simulink model "bh_4bar_model_matrix_VEL_ANALYSIS"  (R2020b)
settings: Solver=ode45  StartTime=0.0  StopTime=2.0944  MaxStep=0.1  RelTol=1e-5  EnableMultiTasking=on
values from neighbouring files (symbols this model uses):
  N = length(THE_DEG_ANG_VEC)    [bh_4bar_kin_z_analysis_CLS.m]
  X = my_stuff_T.theta_deg_vec    [bh_4bar_kin_z_analysis_CLS.m]
undefined symbols (not defined in the file or in its folder): H, my_L1, my_L2, my_L3, theta_0_rad, theta_dot_0_rad, W, Y, Z
libraries: nesl_utility x27, sm_lib x19, simulink_extras x10, simulink x1
settings Model: EnablePacing=on  Creator=bhorton  LastModifiedBy=bhorton
settings DataIOCC: LimitDataPoints=on  ReturnWorkspaceOutputs=off
settings OptimizationCC: LifeSpan=inf
settings DebuggingCC: AllowSymbolicDim=off  PregeneratedLibrarySubsystemCodeDiagnostic=none  SFUnexpectedBacktrackingDiag=warning  SFNoUnconditionalDefaultTransitionDiag=warning  SFExecutionAtInitializationDiag=none  ArithmeticOperatorsInVariantConditions=warning
settings SFSimCC: SimUseLocalCustomCode=off  CustomCodeUndefinedFunction=UseInterfaceOnly
settings RTWCC: RTWUseLocalCustomCode=off
settings CodeAppCC: StateflowObjectComments=on
settings GRTTargetCC: TargetLangStandard=C89/C90 (ANSI)
settings ConfigComp: CovMetricSettings=dw  CovSaveCumulativeToWorkspaceVar=on  CovSaveSingleToWorkspaceVar=on  CovExternalEMLEnable=off  CovSFcnEnable=off
settings SimscapeCC: SimscapeNominalValues="[{\"value\":\"10\",\"unit\":\"V\"},{\"value\":\"1\",\"unit\":\"A\"},{\"value\":\"10\",\"unit\":\"N*m\"},{\"value\":\"10\",\"unit\":\"bar\"},{\"value\":\"100\",\"unit\":\"kJ/kg\"},{\"value\":\"1\",\"unit\":\"kW\"},{\"value\":\"300\",\"unit\":\"K\"},{\"value\":\"100\",\"unit\":\"cm^3/s\"},{\"value\":\"1\",\"unit\":\"kN\"},{\"value\":\"1\",\"unit\":\"g/cm^3\"},{\"value\":\"1\",\"unit\":\"l\"},{\"value\":\"1\",\"unit\":\"cm^2\"},{\"value\":\"60\",\"unit\":\"Hz\"}]"  SimscapeLogType=all  SimscapeLogDataHistory=10000
settings ConfigurationSet: Description=SimMechanics 2G
settings ExplorerConfigSet: InternalSimMechanicsExplorerSettings="<ExplorerConfiguration><canonicalview>default</canonicalview><AnimationSetting><BasePlaybackSpeed>1.0</BasePlaybackSpeed><PlaybackSpeedFactor>1.0</PlaybackSpeedFactor></AnimationSetting><TilePanel><TileInfo><Tiles Columns=\"1\" Count=\"1\" Rows=\"1\"><Column Weight=\"1\"/><Row Weight=\"1\"/><Tile Height=\"1\" Width=\"1\" X=\"0\" Y=\"0\"/></Tiles></TileInfo><SceneInfo><SceneViewer><BGColor><R>0.60000002384185791</R><G>0.60000002384185791</G><B>0.60000002384185791</B></BGColor><Camera><DoPerspective>off</DoPerspective><Position><X>0.48098260470042925</X><Y>0.18774551148408275</Y><Z>1.11774542835223722</Z></Position><Center><X>0.48098260470042925</X><Y>0.18774551148408275</Y><Z>-0.00200006458294343936</Z></Center><Up><X>0</X><Y>1</Y><Z>-0</Z></Up><ViewLimDist>1</ViewLimDist><YLim>0.629325279208176824</YLim><XLim>0.925807410746251169</XLim></Camera></SceneViewer></SceneInfo></TilePanel><MechEditorPanel><Cameras/><GfxPanelCameraMap/><VideoCreator><PlaybackSpeedRatio>0.25</PlaybackSpeedRatio><FrameRate>30</FrameRate><VideoFormat>Motion JPEG AVI</VideoFormat><FrameSize>auto</FrameSize></VideoCreator></MechEditorPanel></ExplorerConfiguration>"

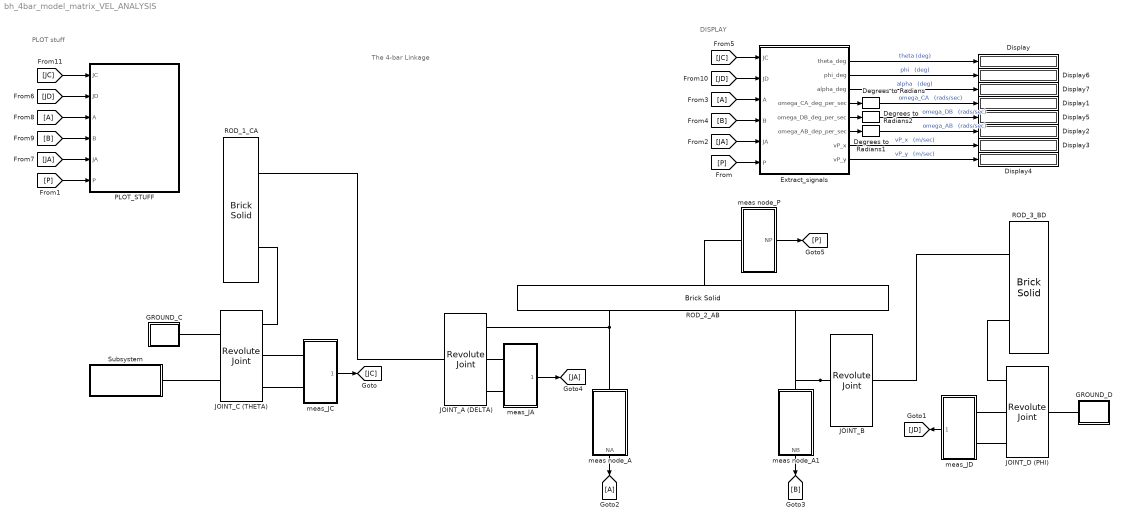
== system bh_4bar_model_matrix_VEL_ANALYSIS ==
  note: DISPLAY
  note: PLOT stuff
  note: The 4-bar Linkage
  Degrees to Radians : simulink_extras/Transformations/Degrees to Radians
  Degrees to Radians1 : simulink_extras/Transformations/Degrees to Radians
  Degrees to Radians2 : simulink_extras/Transformations/Degrees to Radians
  Display{,1..7} (8 alike) : Display
  Extract_signals : Subsystem
  GROUND_C : Subsystem
  GROUND_D : Subsystem
  JOINT_A (DELTA) : sm_lib/Joints/Revolute Joint  JointMode=Normal  SenseConstraintForce=off  SenseConstraintForceX=off  SenseConstraintForceY=off  SenseConstraintForceZ=off  SenseConstraintTorque=off  SenseConstraintTorqueX=off  SenseConstraintTorqueY=off  SenseConstraintTorqueZ=off  SenseTotalForce=off  SenseTotalForceX=off  SenseTotalForceY=off  SenseTotalForceZ=off  SenseTotalTorque=off  SenseTotalTorqueX=off  SenseTotalTorqueY=off  SenseTotalTorqueZ=off  CompositeWrenchDir=FollowerOnBase  CompositeWrenchFrame=BaseFrame  EquilibriumPosition=0  EquilibriumPositionUnits=deg  SpringStiffness=0  SpringStiffnessUnits=N*m/deg  DampingCoefficient=0  DampingCoefficientUnits=N*m/(deg/s)  TorqueActuationMode=NoTorque  MotionActuationMode=ComputedMotion  SensePosition=on  SenseVelocity=on  SenseAcceleration=off  SenseTorqueForce=off  SenseLowerLimitTorqueForce=off  SenseUpperLimitTorqueForce=off  LowerLimitSpecify=off  LowerLimitBound=-90  LowerLimitBoundUnits=deg  LowerLimitStiffness=1e4  LowerLimitStiffnessUnits=N*m/deg  LowerLimitDamping=10  LowerLimitDampingUnits=N*m/(deg/s)  LowerLimitTransitionRegionWidth=0.1  LowerLimitTransitionRegionWidthUnits=deg  UpperLimitSpecify=off  UpperLimitBound=90  UpperLimitBoundUnits=deg  UpperLimitStiffness=1e4  UpperLimitStiffnessUnits=N*m/deg  UpperLimitDamping=10  UpperLimitDampingUnits=N*m/(deg/s)  UpperLimitTransitionRegionWidth=0.1  UpperLimitTransitionRegionWidthUnits=deg  PositionTargetSpecify=off  PositionTargetPriority=High  PositionTargetValue=0  PositionTargetValueUnits=deg  VelocityTargetSpecify=off  VelocityTargetPriority=High  VelocityTargetValue=0  VelocityTargetValueUnits=deg/s
  JOINT_B : sm_lib/Joints/Revolute Joint  JointMode=Normal  SenseConstraintForce=off  SenseConstraintForceX=off  SenseConstraintForceY=off  SenseConstraintForceZ=off  SenseConstraintTorque=off  SenseConstraintTorqueX=off  SenseConstraintTorqueY=off  SenseConstraintTorqueZ=off  SenseTotalForce=off  SenseTotalForceX=off  SenseTotalForceY=off  SenseTotalForceZ=off  SenseTotalTorque=off  SenseTotalTorqueX=off  SenseTotalTorqueY=off  SenseTotalTorqueZ=off  CompositeWrenchDir=FollowerOnBase  CompositeWrenchFrame=BaseFrame  EquilibriumPosition=0  EquilibriumPositionUnits=deg  SpringStiffness=0  SpringStiffnessUnits=N*m/deg  DampingCoefficient=0  DampingCoefficientUnits=N*m/(deg/s)  TorqueActuationMode=NoTorque  MotionActuationMode=ComputedMotion  SensePosition=off  SenseVelocity=off  SenseAcceleration=off  SenseTorqueForce=off  SenseLowerLimitTorqueForce=off  SenseUpperLimitTorqueForce=off  LowerLimitSpecify=off  LowerLimitBound=-90  LowerLimitBoundUnits=deg  LowerLimitStiffness=1e4  LowerLimitStiffnessUnits=N*m/deg  LowerLimitDamping=10  LowerLimitDampingUnits=N*m/(deg/s)  LowerLimitTransitionRegionWidth=0.1  LowerLimitTransitionRegionWidthUnits=deg  UpperLimitSpecify=off  UpperLimitBound=90  UpperLimitBoundUnits=deg  UpperLimitStiffness=1e4  UpperLimitStiffnessUnits=N*m/deg  UpperLimitDamping=10  UpperLimitDampingUnits=N*m/(deg/s)  UpperLimitTransitionRegionWidth=0.1  UpperLimitTransitionRegionWidthUnits=deg  PositionTargetSpecify=off  PositionTargetPriority=High  PositionTargetValue=0  PositionTargetValueUnits=deg  VelocityTargetSpecify=off  VelocityTargetPriority=High  VelocityTargetValue=0  VelocityTargetValueUnits=deg/s
  JOINT_C (THETA) : sm_lib/Joints/Revolute Joint  JointMode=Normal  SenseConstraintForce=off  SenseConstraintForceX=off  SenseConstraintForceY=off  SenseConstraintForceZ=off  SenseConstraintTorque=off  SenseConstraintTorqueX=off  SenseConstraintTorqueY=off  SenseConstraintTorqueZ=off  SenseTotalForce=off  SenseTotalForceX=off  SenseTotalForceY=off  SenseTotalForceZ=off  SenseTotalTorque=off  SenseTotalTorqueX=off  SenseTotalTorqueY=off  SenseTotalTorqueZ=off  CompositeWrenchDir=FollowerOnBase  CompositeWrenchFrame=BaseFrame  EquilibriumPosition=0  EquilibriumPositionUnits=deg  SpringStiffness=0  SpringStiffnessUnits=N*m/deg  DampingCoefficient=0  DampingCoefficientUnits=N*m/(deg/s)  TorqueActuationMode=ComputedTorque  MotionActuationMode=InputMotion  SensePosition=on  SenseVelocity=on  SenseAcceleration=off  SenseTorqueForce=off  SenseLowerLimitTorqueForce=off  SenseUpperLimitTorqueForce=off  LowerLimitSpecify=off  LowerLimitBound=-90  LowerLimitBoundUnits=deg  LowerLimitStiffness=1e4  LowerLimitStiffnessUnits=N*m/deg  LowerLimitDamping=10  LowerLimitDampingUnits=N*m/(deg/s)  LowerLimitTransitionRegionWidth=0.1  LowerLimitTransitionRegionWidthUnits=deg  UpperLimitSpecify=off  UpperLimitBound=90  UpperLimitBoundUnits=deg  UpperLimitStiffness=1e4  UpperLimitStiffnessUnits=N*m/deg  UpperLimitDamping=10  UpperLimitDampingUnits=N*m/(deg/s)  UpperLimitTransitionRegionWidth=0.1  UpperLimitTransitionRegionWidthUnits=deg  PositionTargetSpecify=on  PositionTargetPriority=High  PositionTargetValue=joints.C.ang_degs  PositionTargetValueUnits=deg  VelocityTargetSpecify=on  VelocityTargetPriority=High  VelocityTargetValue=joints.C.vel_degs  VelocityTargetValueUnits=deg/s
      settings: AttributesFormatString=|
      | init_pos =%<PositionTargetValue>
      | %<PositionTargetValueUnits>
      | int_vel = %<VelocityTargetValue>
      | %<VelocityTargetValueUnits>
  JOINT_D (PHI) : sm_lib/Joints/Revolute Joint  JointMode=Normal  SenseConstraintForce=off  SenseConstraintForceX=off  SenseConstraintForceY=off  SenseConstraintForceZ=off  SenseConstraintTorque=off  SenseConstraintTorqueX=off  SenseConstraintTorqueY=off  SenseConstraintTorqueZ=off  SenseTotalForce=off  SenseTotalForceX=off  SenseTotalForceY=off  SenseTotalForceZ=off  SenseTotalTorque=off  SenseTotalTorqueX=off  SenseTotalTorqueY=off  SenseTotalTorqueZ=off  CompositeWrenchDir=FollowerOnBase  CompositeWrenchFrame=BaseFrame  EquilibriumPosition=0  EquilibriumPositionUnits=deg  SpringStiffness=0  SpringStiffnessUnits=N*m/deg  DampingCoefficient=0  DampingCoefficientUnits=N*m/(deg/s)  TorqueActuationMode=NoTorque  MotionActuationMode=ComputedMotion  SensePosition=on  SenseVelocity=on  SenseAcceleration=off  SenseTorqueForce=off  SenseLowerLimitTorqueForce=off  SenseUpperLimitTorqueForce=off  LowerLimitSpecify=off  LowerLimitBound=-90  LowerLimitBoundUnits=deg  LowerLimitStiffness=1e4  LowerLimitStiffnessUnits=N*m/deg  LowerLimitDamping=10  LowerLimitDampingUnits=N*m/(deg/s)  LowerLimitTransitionRegionWidth=0.1  LowerLimitTransitionRegionWidthUnits=deg  UpperLimitSpecify=off  UpperLimitBound=90  UpperLimitBoundUnits=deg  UpperLimitStiffness=1e4  UpperLimitStiffnessUnits=N*m/deg  UpperLimitDamping=10  UpperLimitDampingUnits=N*m/(deg/s)  UpperLimitTransitionRegionWidth=0.1  UpperLimitTransitionRegionWidthUnits=deg  PositionTargetSpecify=on  PositionTargetPriority=High  PositionTargetValue=joints.D.ang_degs  PositionTargetValueUnits=deg  VelocityTargetSpecify=off  VelocityTargetPriority=High  VelocityTargetValue=0  VelocityTargetValueUnits=deg/s
      settings: AttributesFormatString=|
      | init_pos =%<PositionTargetValue>
      | %<PositionTargetValueUnits>
  PLOT_STUFF : Subsystem
  ROD_1_CA : sm_lib/Body Elements/Brick Solid  GraphicAmbientColor=[0.15 0.15 0.15 1.0]  BasedOnType=Density  BrickDimensions=[my_L1,H,W]  BrickDimensionUnits=m  CenterOfMass=[0 0 0]  CenterOfMassUnits=m  GraphicDiffuseColor=[1.0 0.4 0.6]  Density=density  DensityUnits=kg/m^3  DoExposeReferenceFrame=on  GraphicEmissiveColor=[0.0 0.0 0.0 1.0]  ExportEntireGeometry=off  SerializedFrames=<Frames><Frame><Id>Frame2</Id><Value><Name>A</Name><Origin><Source>GeometricFeature</Source><FeatureName>+z +x curve</FeatureName></Origin><PrimaryAxis><DefinedDirection>+Z</DefinedDirection><Source>ReferenceFrame</Source><SourceDirection>+Z</SourceDirection><FeatureName></FeatureName></PrimaryAxis><SecondaryAxis><DefinedDirection>+X</DefinedDirection><Source>ReferenceFrame</Source><SourceDirection>+X</SourceDirection><FeatureName></FeatureName></SecondaryAxis></Value></Frame><Frame><Id>Frame3</Id><Value><Name>C</Name><Origin><Source>GeometricFeature</Source><FeatureName>+z -x curve</FeatureName></Origin><PrimaryAxis><DefinedDirection>+Z</DefinedDirection><Source>ReferenceFrame</Source><SourceDirection>+Z</SourceDirection><FeatureName></FeatureName></PrimaryAxis><SecondaryAxis><DefinedDirection>+X</DefinedDirection><Source>ReferenceFrame</Source><SourceDirection>+X</SourceDirection><FeatureName></FeatureName></SecondaryAxis></Value></Frame></Frames>  MarkerShape=Sphere  MarkerSize=10  GraphicType=FromGeometry  InertiaType=CalculateFromGeometry  Mass=1  MassUnits=kg  MomentsOfInertia=[1 1 1]  MomentsOfInertiaUnits=kg*m^2  GraphicOpacity=1.0  ProductsOfInertia=[0 0 0]  ProductsOfInertiaUnits=kg*m^2  GraphicShininess=75  GraphicSpecularColor=[0.5 0.5 0.5 1.0]  GraphicVisPropType=SimpleVisualProperties
  ROD_2_AB : sm_lib/Body Elements/Brick Solid  GraphicAmbientColor=[0.15 0.15 0.15 1.0]  BasedOnType=Density  BrickDimensions=[my_L2,H,W]  BrickDimensionUnits=m  CenterOfMass=[0 0 0]  CenterOfMassUnits=m  GraphicDiffuseColor=[0.0 1.0 0.2]  Density=density  DensityUnits=kg/m^3  DoExposeReferenceFrame=on  GraphicEmissiveColor=[0.0 0.0 0.0 1.0]  ExportEntireGeometry=off  SerializedFrames=<Frames><Frame><Id>Frame1</Id><Value><Name>A</Name><Origin><Source>GeometricFeature</Source><FeatureName>+z -x curve</FeatureName></Origin><PrimaryAxis><DefinedDirection>+Z</DefinedDirection><Source>ReferenceFrame</Source><SourceDirection>+Z</SourceDirection><FeatureName></FeatureName></PrimaryAxis><SecondaryAxis><DefinedDirection>+X</DefinedDirection><Source>ReferenceFrame</Source><SourceDirection>+X</SourceDirection><FeatureName></FeatureName></SecondaryAxis></Value></Frame><Frame><Id>Frame2</Id><Value><Name>B</Name><Origin><Source>GeometricFeature</Source><FeatureName>+z +x curve</FeatureName></Origin><PrimaryAxis><DefinedDirection>+Z</DefinedDirection><Source>ReferenceFrame</Source><SourceDirection>+Z</SourceDirection><FeatureName></FeatureName></PrimaryAxis><SecondaryAxis><DefinedDirection>+X</DefinedDirection><Source>ReferenceFrame</Source><SourceDirection>+X</SourceDirection><FeatureName></FeatureName></SecondaryAxis></Value></Frame></Frames>  MarkerShape=Sphere  MarkerSize=10  GraphicType=FromGeometry  InertiaType=CalculateFromGeometry  Mass=1  MassUnits=kg  MomentsOfInertia=[1 1 1]  MomentsOfInertiaUnits=kg*m^2  GraphicOpacity=1.0  ProductsOfInertia=[0 0 0]  ProductsOfInertiaUnits=kg*m^2  GraphicShininess=75  GraphicSpecularColor=[0.5 0.5 0.5 1.0]  GraphicVisPropType=SimpleVisualProperties
  ROD_3_BD : sm_lib/Body Elements/Brick Solid  GraphicAmbientColor=[0.15 0.15 0.15 1.0]  BasedOnType=Density  BrickDimensions=[my_L3,H,W]  BrickDimensionUnits=m  CenterOfMass=[0 0 0]  CenterOfMassUnits=m  GraphicDiffuseColor=[0.2 0.2 1.0]  Density=density  DensityUnits=kg/m^3  DoExposeReferenceFrame=on  GraphicEmissiveColor=[0.0 0.0 0.0 1.0]  ExportEntireGeometry=off  SerializedFrames=<Frames><Frame><Id>Frame1</Id><Value><Name>B</Name><Origin><Source>GeometricFeature</Source><FeatureName>+z +x curve</FeatureName></Origin><PrimaryAxis><DefinedDirection>+Z</DefinedDirection><Source>ReferenceFrame</Source><SourceDirection>+Z</SourceDirection><FeatureName></FeatureName></PrimaryAxis><SecondaryAxis><DefinedDirection>+X</DefinedDirection><Source>ReferenceFrame</Source><SourceDirection>+X</SourceDirection><FeatureName></FeatureName></SecondaryAxis></Value></Frame><Frame><Id>Frame2</Id><Value><Name>D</Name><Origin><Source>GeometricFeature</Source><FeatureName>+z -x curve</FeatureName></Origin><PrimaryAxis><DefinedDirection>+Z</DefinedDirection><Source>ReferenceFrame</Source><SourceDirection>+Z</SourceDirection><FeatureName></FeatureName></PrimaryAxis><SecondaryAxis><DefinedDirection>+X</DefinedDirection><Source>ReferenceFrame</Source><SourceDirection>+X</SourceDirection><FeatureName></FeatureName></SecondaryAxis></Value></Frame></Frames>  MarkerShape=Sphere  MarkerSize=10  GraphicType=FromGeometry  InertiaType=CalculateFromGeometry  Mass=1  MassUnits=kg  MomentsOfInertia=[1 1 1]  MomentsOfInertiaUnits=kg*m^2  GraphicOpacity=1.0  ProductsOfInertia=[0 0 0]  ProductsOfInertiaUnits=kg*m^2  GraphicShininess=75  GraphicSpecularColor=[0.5 0.5 0.5 1.0]  GraphicVisPropType=SimpleVisualProperties
  Subsystem : Subsystem
  meas node_A : Subsystem
      mask Display: image('$imagefile'); % Use "Edit Image" on toolstrip to change.
  meas node_A1 : Subsystem
      mask Display: image('$imagefile'); % Use "Edit Image" on toolstrip to change.
  meas node_P : Subsystem
      mask Display: image('$imagefile'); % Use "Edit Image" on toolstrip to change.
  meas_JA : Subsystem
      mask Display: image('$imagefile'); % Use "Edit Image" on toolstrip to change.
  meas_JC : Subsystem
      mask Display: image('$imagefile'); % Use "Edit Image" on toolstrip to change.
  meas_JD : Subsystem
      mask Display: image('$imagefile'); % Use "Edit Image" on toolstrip to change.
  wires:
  meas node_A1/1(NB) -> [B]
  meas_JA/1(PV_BUS) -> [JA]
  meas_JD/1(PV_BUS) -> [JD]
  meas_JC/1(PV_BUS) -> [JC]
  meas node_A/1(NA) -> [A]
  meas node_P/1(NP) -> [P]
  [JC] -> Extract_signals/1(JC)
  [JA] -> Extract_signals/5(JA)
  Extract_signals/1(theta_deg) -> Display/1  "theta (deg)"
  [B] -> Extract_signals/4(B)
  Extract_signals/8(vP_y) -> Display4/1  "vP_y   (m/sec)"
  [A] -> Extract_signals/3(A)
  Extract_signals/7(vP_x) -> Display3/1  "vP_x   (m/sec)"
  Degrees to Radians/1 -> Display1/1  "omega_CA   (rads/sec)"
  Degrees to Radians1/1 -> Display2/1  "omega_AB   (rads/sec)"
  [P] -> Extract_signals/6(P)
  [JD] -> Extract_signals/2(JD)
  Extract_signals/6(omega_AB_dep_per_sec) -> Degrees to Radians1/1
  Extract_signals/4(omega_CA_deg_per_sec) -> Degrees to Radians/1
  Extract_signals/5(omega_DB_deg_per_sec) -> Degrees to Radians2/1
  Degrees to Radians2/1 -> Display5/1  "omega_DB   (rads/sec)"
  Extract_signals/2(phi_deg) -> Display6/1  "phi   (deg)"
  Extract_signals/3(alpha_deg) -> Display7/1  "alpha   (deg)"
  [JC] -> PLOT_STUFF/1(JC)
  [JD] -> PLOT_STUFF/2(JD)
  [A] -> PLOT_STUFF/3(A)
  [B] -> PLOT_STUFF/4(B)
  [JA] -> PLOT_STUFF/5(JA)
  [P] -> PLOT_STUFF/6(P)
  connections:
  meas node_A/LConn1 -- JOINT_A (DELTA)/RConn1 -- ROD_2_AB/LConn1
  JOINT_B/LConn1 -- meas node_A1/LConn1 -- ROD_2_AB/LConn2
  meas_JA/LConn2 -- JOINT_A (DELTA)/RConn3
  meas_JD/LConn1 -- JOINT_D (PHI)/RConn2
  meas_JA/LConn1 -- JOINT_A (DELTA)/RConn2
  JOINT_C (THETA)/RConn1 -- ROD_1_CA/LConn2
  JOINT_C (THETA)/RConn3 -- meas_JC/LConn2
  ROD_3_BD/LConn1 -- JOINT_B/RConn1
  GROUND_D/RConn1 -- JOINT_D (PHI)/LConn1
  JOINT_C (THETA)/LConn1 -- GROUND_C/RConn1
  JOINT_D (PHI)/RConn1 -- ROD_3_BD/LConn2
  meas_JD/LConn2 -- JOINT_D (PHI)/RConn3
  JOINT_C (THETA)/RConn2 -- meas_JC/LConn1
  ROD_1_CA/LConn1 -- JOINT_A (DELTA)/LConn1
  meas node_P/LConn1 -- ROD_2_AB/RConn1
  Subsystem/LConn1 -- JOINT_C (THETA)/LConn2

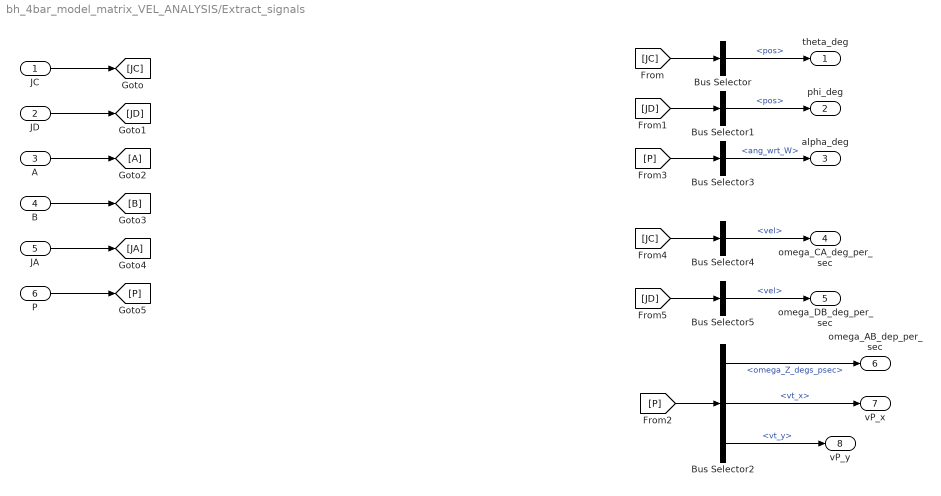
== system bh_4bar_model_matrix_VEL_ANALYSIS/Extract_signals ==
  JC : Inport
  JD : Inport  Port=2
  A : Inport  Port=3
  B : Inport  Port=4
  JA : Inport  Port=5
  P : Inport  Port=6
  Bus Selector : BusSelector  OutputSignals=pos
  Bus Selector1 : BusSelector  OutputSignals=pos
  Bus Selector2 : BusSelector  OutputSignals=omega_Z_degs_psec,vt_x,vt_y
  Bus Selector3 : BusSelector  OutputSignals=ang_wrt_W
  Bus Selector4 : BusSelector  OutputSignals=vel
  Bus Selector5 : BusSelector  OutputSignals=vel
  theta_deg : Outport  VectorParamsAs1DForOutWhenUnconnected=off
  phi_deg : Outport  Port=2  VectorParamsAs1DForOutWhenUnconnected=off
  alpha_deg : Outport  Port=3  VectorParamsAs1DForOutWhenUnconnected=off
  omega_CA_deg_per_sec : Outport  Port=4  VectorParamsAs1DForOutWhenUnconnected=off
  omega_DB_deg_per_sec : Outport  Port=5  VectorParamsAs1DForOutWhenUnconnected=off
  omega_AB_dep_per_sec : Outport  Port=6  VectorParamsAs1DForOutWhenUnconnected=off
  vP_x : Outport  Port=7  VectorParamsAs1DForOutWhenUnconnected=off
  vP_y : Outport  Port=8  VectorParamsAs1DForOutWhenUnconnected=off
  wires:
  B/1 -> [B]
  A/1 -> [A]
  JD/1 -> [JD]
  JC/1 -> [JC]
  [JC] -> Bus Selector/1
  JA/1 -> [JA]
  P/1 -> [P]
  Bus Selector/1 -> theta_deg/1  "<pos>"
  Bus Selector4/1 -> omega_CA_deg_per_sec/1  "<vel>"
  [P] -> Bus Selector2/1
  Bus Selector2/1 -> omega_AB_dep_per_sec/1  "<omega_Z_degs_psec>"
  Bus Selector2/2 -> vP_x/1  "<vt_x>"
  Bus Selector2/3 -> vP_y/1  "<vt_y>"
  [JD] -> Bus Selector1/1
  Bus Selector1/1 -> phi_deg/1  "<pos>"
  [P] -> Bus Selector3/1
  Bus Selector3/1 -> alpha_deg/1  "<ang_wrt_W>"
  [JC] -> Bus Selector4/1
  Bus Selector5/1 -> omega_DB_deg_per_sec/1  "<vel>"
  [JD] -> Bus Selector5/1

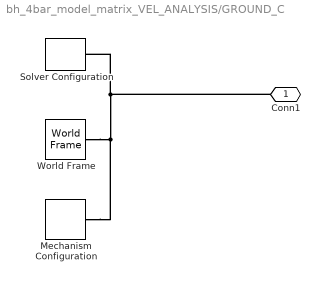
== system bh_4bar_model_matrix_VEL_ANALYSIS/GROUND_C ==
  Mechanism Configuration : sm_lib/Utilities/Mechanism Configuration  UniformGravity=Constant  GravityVector=[0 0 0]  GravityVectorUnits=m/s^2  GravityUnits=m/s^2  LinearizationDelta=0.001  JointModeTransitionNonlinearIterations=2
  Solver Configuration : nesl_utility/Solver Configuration  PhysicalDomain=network_engine_domain  SubClassName=solver  LeftPortType=input  RightPortType=generic  Tones=[]  Harmonics=[]  SimulateNoise=off  Profile=off  UseLocalSampling=off  EnableSwitchedLinearOptims=on  FrequencyDomain=off  UseCCode=off  RelTol=0.001  AbsTol=1e-06  MinStep=1e-09  ToWorkspace=off  RevertToSquareIcSolve=off  NumHomotopyIterations=100  PhasorMode=off  PhasorModeNumHarmonics=1  DoDC=off  ResidualTolerance=1e-09  UseLocalSolver=off  LocalSolverChoice=NE_BACKWARD_EULER_ADVANCER  LocalSolverSampleTime=0.001  DoFixedCost=off  MaxNonlinIter=3  MaxModeIter=2  ComputeImpulses=off  ImpulseIterations=2  LinearAlgebra=Sparse  EquationFormulation=NE_TIME_EF  DelaysMemoryBudget=1024  AutomaticFiltering=on  FilteringTimeConstant=0.001  PartitionStorageMethod=AS_NEEDED  PartitionMemoryBudget=1024  PartitionMethod=FAST
  World Frame : sm_lib/Frames and Transforms/World Frame
  Conn1 : PMIOPort  Side=Right
  connections:
  Solver Configuration/RConn1 -- Conn1/RConn1 -- Mechanism Configuration/RConn1 -- World Frame/RConn1

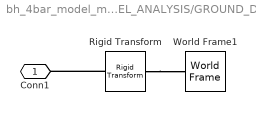
== system bh_4bar_model_matrix_VEL_ANALYSIS/GROUND_D ==
  Rigid Transform : sm_lib/Frames and Transforms/Rigid Transform  TranslationMethod=StandardAxis  TranslationStandardOffset=my_L4  TranslationLengthUnit=m  TranslationStandardAxis=+X  TranslationCartesianOffset=[0 0 0]  TranslationROffset=0  TranslationROffsetUnits=m  TranslationZOffset=0  TranslationZOffsetUnits=m  TranslationThetaOffset=0  TranslationThetaOffsetUnits=deg  RotationMethod=None  RotationAngleUnits=deg  RotationStandardAxis=+Z  RotationAngle=0.0  RotationArbitraryAxis=[0 0 1]  FollAlignAxisA=+X  BaseAlignAxisA=+Y  FollAlignAxisB=+Y  BaseAlignAxisB=+Z  RotationSequenceAxes=FollowerAxes  RotationSequence=XYX  RotationSequenceAngles=[0 0 0]  RotationSequenceAnglesUnits=deg  RotationMatrix=[1 0 0; 0 1 0; 0 0 1]
  World Frame1 : sm_lib/Frames and Transforms/World Frame
  Conn1 : PMIOPort  Side=Right
  connections:
  Rigid Transform/LConn1 -- World Frame1/RConn1
  Rigid Transform/RConn1 -- Conn1/RConn1

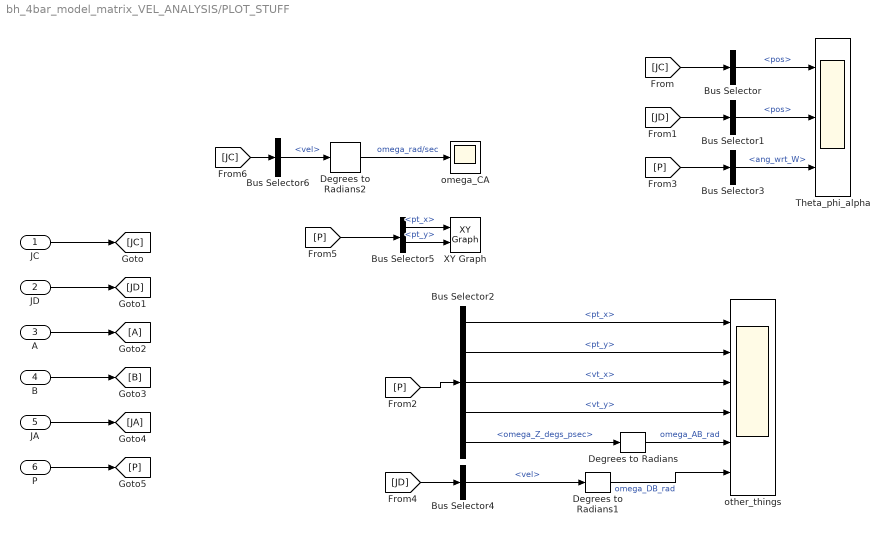
== system bh_4bar_model_matrix_VEL_ANALYSIS/PLOT_STUFF ==
  JC : Inport
  JD : Inport  Port=2
  A : Inport  Port=3
  B : Inport  Port=4
  JA : Inport  Port=5
  P : Inport  Port=6
  Bus Selector : BusSelector  OutputSignals=pos
  Bus Selector1 : BusSelector  OutputSignals=pos
  Bus Selector2 : BusSelector  OutputSignals=pt_x,pt_y,vt_x,vt_y,omega_Z_degs_psec
  Bus Selector3 : BusSelector  OutputSignals=ang_wrt_W
  Bus Selector4 : BusSelector  OutputSignals=vel
  Bus Selector5 : BusSelector  OutputSignals=pt_x,pt_y
  Bus Selector6 : BusSelector  OutputSignals=vel
  Degrees to Radians : simulink_extras/Transformations/Degrees to Radians
  Degrees to Radians1 : simulink_extras/Transformations/Degrees to Radians
  Degrees to Radians2 : simulink_extras/Transformations/Degrees to Radians
  Theta_phi_alpha : Scope  NumInputPorts=3
  XY Graph : simulink/Sinks/XY Graph  xmin=-1  xmax=1  ymin=-1  ymax=1  st=-1
  omega_CA : Scope
  other_things : Scope  NumInputPorts=6
  wires:
  B/1 -> [B]
  A/1 -> [A]
  JD/1 -> [JD]
  JC/1 -> [JC]
  JA/1 -> [JA]
  P/1 -> [P]
  [JC] -> Bus Selector/1
  [JD] -> Bus Selector1/1
  Bus Selector/1 -> Theta_phi_alpha/1  "<pos>"
  Bus Selector1/1 -> Theta_phi_alpha/2  "<pos>"
  [P] -> Bus Selector3/1
  Bus Selector3/1 -> Theta_phi_alpha/3  "<ang_wrt_W>"
  [P] -> Bus Selector2/1
  Bus Selector2/1 -> other_things/1  "<pt_x>"
  Bus Selector2/2 -> other_things/2  "<pt_y>"
  Bus Selector2/3 -> other_things/3  "<vt_x>"
  Bus Selector2/4 -> other_things/4  "<vt_y>"
  Bus Selector2/5 -> Degrees to Radians/1  "<omega_Z_degs_psec>"
  Degrees to Radians/1 -> other_things/5  "omega_AB_rad"
  [JD] -> Bus Selector4/1
  Bus Selector4/1 -> Degrees to Radians1/1  "<vel>"
  Degrees to Radians1/1 -> other_things/6  "omega_DB_rad"
  [P] -> Bus Selector5/1
  Bus Selector5/1 -> XY Graph/1  "<pt_x>"
  Bus Selector5/2 -> XY Graph/2  "<pt_y>"
  [JC] -> Bus Selector6/1
  Bus Selector6/1 -> Degrees to Radians2/1  "<vel>"
  Degrees to Radians2/1 -> omega_CA/1  "omega_rad/sec"

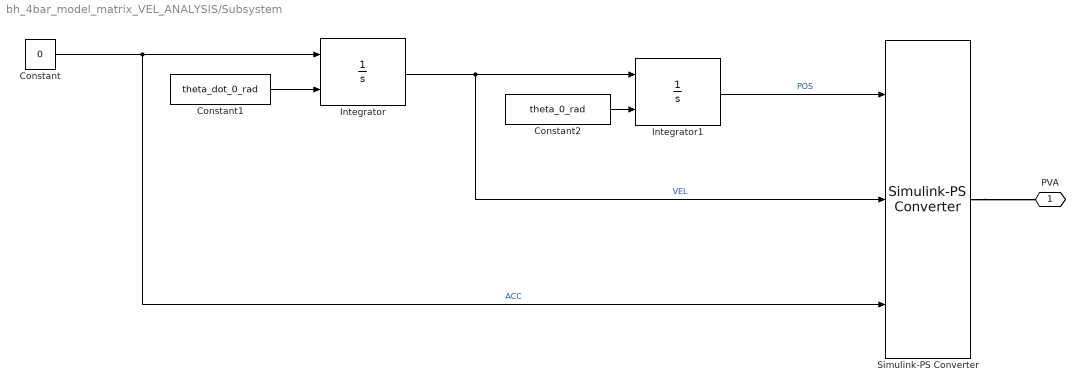
== system bh_4bar_model_matrix_VEL_ANALYSIS/Subsystem ==
  Constant : Constant  Value=0
  Constant1 : Constant  Value=theta_dot_0_rad
  Constant2 : Constant  Value=theta_0_rad
  Integrator : Integrator  InitialConditionSource=external
  Integrator1 : Integrator  InitialConditionSource=external
  Simulink-PS Converter : nesl_utility/Simulink-PS Converter  PhysicalDomain=network_engine_domain  SubClassName=ps_input  LeftPortType=input  RightPortType=output  PseudoPeriodic=off  Frequencies=[]  NoiseDistribution=none  NoiseParameters=[]  Unit=rad  AffineConversion=off  FilteringAndDerivatives=provide  SimscapeFilterOrder=1  InputFilterTimeConstant=0.001  UdotUserProvided=2
      settings: AttributesFormatString=UNITS = %<Unit>
  "PVA " : PMIOPort  Side=Left
  wires:
  Constant2/1 -> Integrator1/2
  Constant/1 -> Simulink-PS Converter/3, Integrator/1  "ACC"
  Constant1/1 -> Integrator/2
  Integrator/1 -> Simulink-PS Converter/2, Integrator1/1  "VEL"
  Integrator1/1 -> Simulink-PS Converter/1  "POS"
  connections:
  Simulink-PS Converter/RConn1 -- "PVA "/RConn1

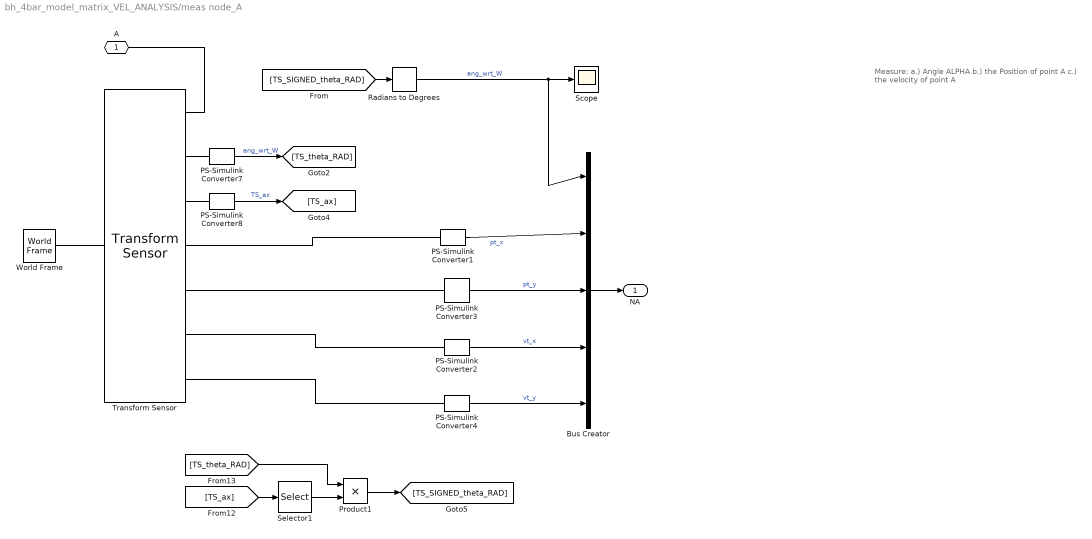
== system bh_4bar_model_matrix_VEL_ANALYSIS/meas node_A ==
  note: Measure:
      | a.) Angle ALPHA
      | b.) the Position of point A
      | c.) the velocity of point A
  Bus Creator : BusCreator  Inputs=5
  PS-Simulink Converter1 : nesl_utility/PS-Simulink Converter  PhysicalDomain=network_engine_domain  SubClassName=ps_output  LeftPortType=input  RightPortType=output  PseudoPeriodic=off  Frequencies=[]  Unit=m  AffineConversion=off
      settings: AttributesFormatString=UNITS=%<Unit>
  PS-Simulink Converter2 : nesl_utility/PS-Simulink Converter  PhysicalDomain=network_engine_domain  SubClassName=ps_output  LeftPortType=input  RightPortType=output  PseudoPeriodic=off  Frequencies=[]  Unit=m/s  AffineConversion=off
      settings: AttributesFormatString=UNITS=%<Unit>
  PS-Simulink Converter3 : nesl_utility/PS-Simulink Converter  PhysicalDomain=network_engine_domain  SubClassName=ps_output  LeftPortType=input  RightPortType=output  PseudoPeriodic=off  Frequencies=[]  Unit=m  AffineConversion=off
      settings: AttributesFormatString=UNITS=%<Unit>
  PS-Simulink Converter4 : nesl_utility/PS-Simulink Converter  PhysicalDomain=network_engine_domain  SubClassName=ps_output  LeftPortType=input  RightPortType=output  PseudoPeriodic=off  Frequencies=[]  Unit=m/s  AffineConversion=off
      settings: AttributesFormatString=UNITS=%<Unit>
  PS-Simulink Converter7 : nesl_utility/PS-Simulink Converter  PhysicalDomain=network_engine_domain  SubClassName=ps_output  LeftPortType=input  RightPortType=output  PseudoPeriodic=off  Frequencies=[]  Unit=rad  AffineConversion=off
      settings: AttributesFormatString=UNITS=%<Unit>
  PS-Simulink Converter8 : nesl_utility/PS-Simulink Converter  PhysicalDomain=network_engine_domain  SubClassName=ps_output  LeftPortType=input  RightPortType=output  PseudoPeriodic=off  Frequencies=[]  Unit=1  AffineConversion=off
      settings: AttributesFormatString=UNITS=%<Unit>
  Product1 : Product
  Radians to Degrees : simulink_extras/Transformations/Radians to Degrees
  Scope : Scope
  Selector1 : Selector  InputPortWidth=3  IndexOptions=Index vector (dialog)  Indices=3  OutputSizes=1
  Transform Sensor : sm_lib/Frames and Transforms/Transform Sensor  MeasurementFrame=World  SenseAngle=on  SenseAxis=on  SenseAngle1=off  SenseAngle2=off  SenseAngle3=off  SenseQ=off  SenseR=off  SenseOmegaX=off  SenseOmegaY=off  SenseOmegaZ=off  SenseOmega1=off  SenseOmega2=off  SenseOmega3=off  SenseQDot=off  SenseRDot=off  SenseAlphaX=off  SenseAlphaY=off  SenseAlphaZ=off  SenseAlpha1=off  SenseAlpha2=off  SenseAlpha3=off  SenseQDDot=off  SenseRDDot=off  SenseX=on  SenseY=on  SenseZ=off  SenseRad=off  SenseAzim=off  SenseDist=off  SenseInc=off  SenseXDot=on  SenseYDot=on  SenseZDot=off  SenseRadDot=off  SenseAzimDot=off  SenseDistDot=off  SenseIncDot=off  SenseXDDot=off  SenseYDDot=off  SenseZDDot=off  SenseRadDDot=off  SenseAzimDDot=off  SenseDistDDot=off  SenseIncDDot=off
  World Frame : sm_lib/Frames and Transforms/World Frame
  A : PMIOPort  Side=Left
  NA : Outport  VectorParamsAs1DForOutWhenUnconnected=off
  wires:
  PS-Simulink Converter2/1 -> Bus Creator/4  "vt_x"
  Bus Creator/1 -> NA/1
  PS-Simulink Converter1/1 -> Bus Creator/2  "pt_x"
  PS-Simulink Converter4/1 -> Bus Creator/5  "vt_y"
  PS-Simulink Converter3/1 -> Bus Creator/3  "pt_y"
  Radians to Degrees/1 -> Bus Creator/1, Scope/1  "ang_wrt_W"
  [TS_theta_RAD] -> Product1/1
  [TS_ax] -> Selector1/1
  Product1/1 -> [TS_SIGNED_theta_RAD]
  Selector1/1 -> Product1/2
  PS-Simulink Converter7/1 -> [TS_theta_RAD]  "ang_wrt_W"
  PS-Simulink Converter8/1 -> [TS_ax]  "TS_ax"
  [TS_SIGNED_theta_RAD] -> Radians to Degrees/1
  connections:
  A/RConn1 -- Transform Sensor/RConn1
  Transform Sensor/LConn1 -- World Frame/RConn1
  Transform Sensor/RConn7 -- PS-Simulink Converter4/LConn1
  PS-Simulink Converter2/LConn1 -- Transform Sensor/RConn6
  PS-Simulink Converter3/LConn1 -- Transform Sensor/RConn5
  PS-Simulink Converter1/LConn1 -- Transform Sensor/RConn4
  PS-Simulink Converter7/LConn1 -- Transform Sensor/RConn2
  PS-Simulink Converter8/LConn1 -- Transform Sensor/RConn3

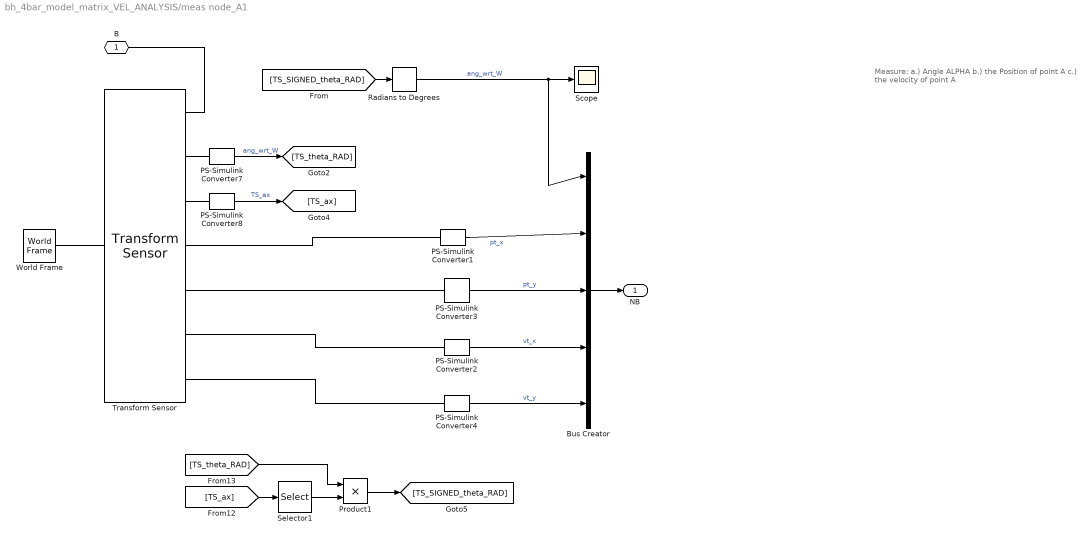
== system bh_4bar_model_matrix_VEL_ANALYSIS/meas node_A1 ==
  note: Measure:
      | a.) Angle ALPHA
      | b.) the Position of point A
      | c.) the velocity of point A
  Bus Creator : BusCreator  Inputs=5
  PS-Simulink Converter1 : nesl_utility/PS-Simulink Converter  PhysicalDomain=network_engine_domain  SubClassName=ps_output  LeftPortType=input  RightPortType=output  PseudoPeriodic=off  Frequencies=[]  Unit=m  AffineConversion=off
      settings: AttributesFormatString=UNITS=%<Unit>
  PS-Simulink Converter2 : nesl_utility/PS-Simulink Converter  PhysicalDomain=network_engine_domain  SubClassName=ps_output  LeftPortType=input  RightPortType=output  PseudoPeriodic=off  Frequencies=[]  Unit=m/s  AffineConversion=off
      settings: AttributesFormatString=UNITS=%<Unit>
  PS-Simulink Converter3 : nesl_utility/PS-Simulink Converter  PhysicalDomain=network_engine_domain  SubClassName=ps_output  LeftPortType=input  RightPortType=output  PseudoPeriodic=off  Frequencies=[]  Unit=m  AffineConversion=off
      settings: AttributesFormatString=UNITS=%<Unit>
  PS-Simulink Converter4 : nesl_utility/PS-Simulink Converter  PhysicalDomain=network_engine_domain  SubClassName=ps_output  LeftPortType=input  RightPortType=output  PseudoPeriodic=off  Frequencies=[]  Unit=m/s  AffineConversion=off
      settings: AttributesFormatString=UNITS=%<Unit>
  PS-Simulink Converter7 : nesl_utility/PS-Simulink Converter  PhysicalDomain=network_engine_domain  SubClassName=ps_output  LeftPortType=input  RightPortType=output  PseudoPeriodic=off  Frequencies=[]  Unit=rad  AffineConversion=off
      settings: AttributesFormatString=UNITS=%<Unit>
  PS-Simulink Converter8 : nesl_utility/PS-Simulink Converter  PhysicalDomain=network_engine_domain  SubClassName=ps_output  LeftPortType=input  RightPortType=output  PseudoPeriodic=off  Frequencies=[]  Unit=1  AffineConversion=off
      settings: AttributesFormatString=UNITS=%<Unit>
  Product1 : Product
  Radians to Degrees : simulink_extras/Transformations/Radians to Degrees
  Scope : Scope
  Selector1 : Selector  InputPortWidth=3  IndexOptions=Index vector (dialog)  Indices=3  OutputSizes=1
  Transform Sensor : sm_lib/Frames and Transforms/Transform Sensor  MeasurementFrame=World  SenseAngle=on  SenseAxis=on  SenseAngle1=off  SenseAngle2=off  SenseAngle3=off  SenseQ=off  SenseR=off  SenseOmegaX=off  SenseOmegaY=off  SenseOmegaZ=off  SenseOmega1=off  SenseOmega2=off  SenseOmega3=off  SenseQDot=off  SenseRDot=off  SenseAlphaX=off  SenseAlphaY=off  SenseAlphaZ=off  SenseAlpha1=off  SenseAlpha2=off  SenseAlpha3=off  SenseQDDot=off  SenseRDDot=off  SenseX=on  SenseY=on  SenseZ=off  SenseRad=off  SenseAzim=off  SenseDist=off  SenseInc=off  SenseXDot=on  SenseYDot=on  SenseZDot=off  SenseRadDot=off  SenseAzimDot=off  SenseDistDot=off  SenseIncDot=off  SenseXDDot=off  SenseYDDot=off  SenseZDDot=off  SenseRadDDot=off  SenseAzimDDot=off  SenseDistDDot=off  SenseIncDDot=off
  World Frame : sm_lib/Frames and Transforms/World Frame
  B : PMIOPort  Side=Left
  NB : Outport  VectorParamsAs1DForOutWhenUnconnected=off
  wires:
  PS-Simulink Converter2/1 -> Bus Creator/4  "vt_x"
  Bus Creator/1 -> NB/1
  PS-Simulink Converter1/1 -> Bus Creator/2  "pt_x"
  PS-Simulink Converter4/1 -> Bus Creator/5  "vt_y"
  PS-Simulink Converter3/1 -> Bus Creator/3  "pt_y"
  Radians to Degrees/1 -> Bus Creator/1, Scope/1  "ang_wrt_W"
  [TS_theta_RAD] -> Product1/1
  [TS_ax] -> Selector1/1
  Product1/1 -> [TS_SIGNED_theta_RAD]
  Selector1/1 -> Product1/2
  PS-Simulink Converter7/1 -> [TS_theta_RAD]  "ang_wrt_W"
  PS-Simulink Converter8/1 -> [TS_ax]  "TS_ax"
  [TS_SIGNED_theta_RAD] -> Radians to Degrees/1
  connections:
  B/RConn1 -- Transform Sensor/RConn1
  Transform Sensor/LConn1 -- World Frame/RConn1
  Transform Sensor/RConn7 -- PS-Simulink Converter4/LConn1
  PS-Simulink Converter2/LConn1 -- Transform Sensor/RConn6
  PS-Simulink Converter3/LConn1 -- Transform Sensor/RConn5
  PS-Simulink Converter1/LConn1 -- Transform Sensor/RConn4
  PS-Simulink Converter7/LConn1 -- Transform Sensor/RConn2
  PS-Simulink Converter8/LConn1 -- Transform Sensor/RConn3

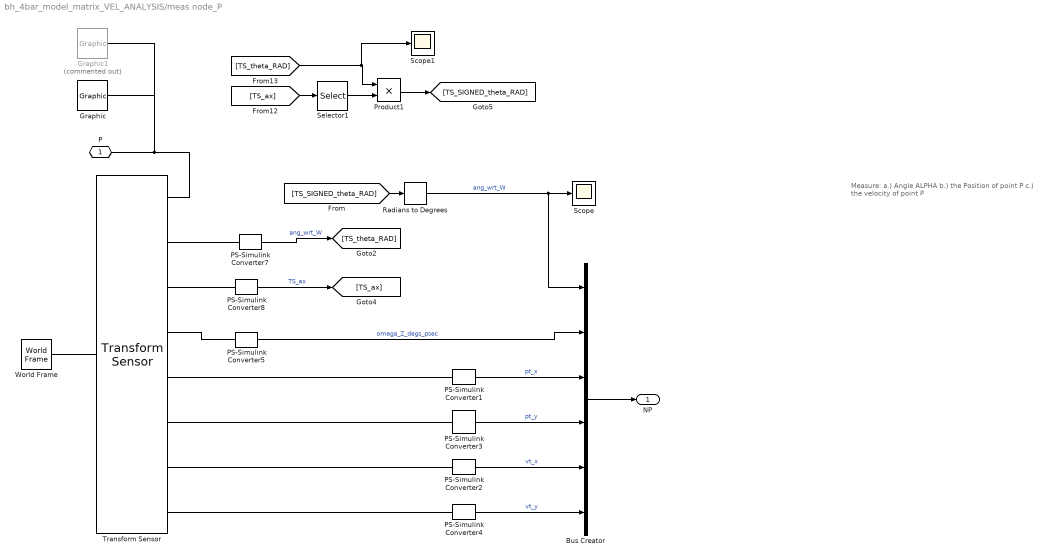
== system bh_4bar_model_matrix_VEL_ANALYSIS/meas node_P ==
  note: Measure:
      | a.) Angle ALPHA
      | b.) the Position of point P
      | c.) the velocity of point P
  Bus Creator : BusCreator  Inputs=6
  Graphic : sm_lib/Body Elements/Graphic  GraphicType=Marker  MarkerShape=Sphere  MarkerSize=20  GraphicVisPropType=SimpleVisualProperties  GraphicDiffuseColor=[0.0 0.0 0.0]  GraphicSpecularColor=[0.5 0.5 0.5 1.0]  GraphicAmbientColor=[0.15 0.15 0.15 1.0]  GraphicEmissiveColor=[0.0 0.0 0.0 1.0]  GraphicShininess=75  GraphicOpacity=1.0
  Graphic1 : sm_lib/Body Elements/Graphic  Commented=on  GraphicType=Marker  MarkerShape=Frame  MarkerSize=33  GraphicVisPropType=SimpleVisualProperties  GraphicDiffuseColor=[0.0 0.0 0.0]  GraphicSpecularColor=[0.5 0.5 0.5 1.0]  GraphicAmbientColor=[0.15 0.15 0.15 1.0]  GraphicEmissiveColor=[0.0 0.0 0.0 1.0]  GraphicShininess=75  GraphicOpacity=1.0
  PS-Simulink Converter1 : nesl_utility/PS-Simulink Converter  PhysicalDomain=network_engine_domain  SubClassName=ps_output  LeftPortType=input  RightPortType=output  PseudoPeriodic=off  Frequencies=[]  Unit=m  AffineConversion=off
      settings: AttributesFormatString=UNITS=%<Unit>
  PS-Simulink Converter2 : nesl_utility/PS-Simulink Converter  PhysicalDomain=network_engine_domain  SubClassName=ps_output  LeftPortType=input  RightPortType=output  PseudoPeriodic=off  Frequencies=[]  Unit=m/s  AffineConversion=off
      settings: AttributesFormatString=UNITS=%<Unit>
  PS-Simulink Converter3 : nesl_utility/PS-Simulink Converter  PhysicalDomain=network_engine_domain  SubClassName=ps_output  LeftPortType=input  RightPortType=output  PseudoPeriodic=off  Frequencies=[]  Unit=m  AffineConversion=off
      settings: AttributesFormatString=UNITS=%<Unit>
  PS-Simulink Converter4 : nesl_utility/PS-Simulink Converter  PhysicalDomain=network_engine_domain  SubClassName=ps_output  LeftPortType=input  RightPortType=output  PseudoPeriodic=off  Frequencies=[]  Unit=m/s  AffineConversion=off
      settings: AttributesFormatString=UNITS=%<Unit>
  PS-Simulink Converter5 : nesl_utility/PS-Simulink Converter  PhysicalDomain=network_engine_domain  SubClassName=ps_output  LeftPortType=input  RightPortType=output  PseudoPeriodic=off  Frequencies=[]  Unit=deg/s  AffineConversion=off
      settings: AttributesFormatString=UNITS=%<Unit>
  PS-Simulink Converter7 : nesl_utility/PS-Simulink Converter  PhysicalDomain=network_engine_domain  SubClassName=ps_output  LeftPortType=input  RightPortType=output  PseudoPeriodic=off  Frequencies=[]  Unit=rad  AffineConversion=off
      settings: AttributesFormatString=UNITS=%<Unit>
  PS-Simulink Converter8 : nesl_utility/PS-Simulink Converter  PhysicalDomain=network_engine_domain  SubClassName=ps_output  LeftPortType=input  RightPortType=output  PseudoPeriodic=off  Frequencies=[]  Unit=1  AffineConversion=off
      settings: AttributesFormatString=UNITS=%<Unit>
  Product1 : Product
  Radians to Degrees : simulink_extras/Transformations/Radians to Degrees
  Scope : Scope
  Scope1 : Scope
  Selector1 : Selector  InputPortWidth=3  IndexOptions=Index vector (dialog)  Indices=3  OutputSizes=1
  Transform Sensor : sm_lib/Frames and Transforms/Transform Sensor  MeasurementFrame=World  SenseAngle=on  SenseAxis=on  SenseAngle1=off  SenseAngle2=off  SenseAngle3=off  SenseQ=off  SenseR=off  SenseOmegaX=off  SenseOmegaY=off  SenseOmegaZ=on  SenseOmega1=off  SenseOmega2=off  SenseOmega3=off  SenseQDot=off  SenseRDot=off  SenseAlphaX=off  SenseAlphaY=off  SenseAlphaZ=off  SenseAlpha1=off  SenseAlpha2=off  SenseAlpha3=off  SenseQDDot=off  SenseRDDot=off  SenseX=on  SenseY=on  SenseZ=off  SenseRad=off  SenseAzim=off  SenseDist=off  SenseInc=off  SenseXDot=on  SenseYDot=on  SenseZDot=off  SenseRadDot=off  SenseAzimDot=off  SenseDistDot=off  SenseIncDot=off  SenseXDDot=off  SenseYDDot=off  SenseZDDot=off  SenseRadDDot=off  SenseAzimDDot=off  SenseDistDDot=off  SenseIncDDot=off
  World Frame : sm_lib/Frames and Transforms/World Frame
  P : PMIOPort  Side=Left
  NP : Outport  VectorParamsAs1DForOutWhenUnconnected=off
  wires:
  PS-Simulink Converter2/1 -> Bus Creator/5  "vt_x"
  Bus Creator/1 -> NP/1
  PS-Simulink Converter1/1 -> Bus Creator/3  "pt_x"
  PS-Simulink Converter4/1 -> Bus Creator/6  "vt_y"
  PS-Simulink Converter3/1 -> Bus Creator/4  "pt_y"
  Radians to Degrees/1 -> Bus Creator/1, Scope/1  "ang_wrt_W"
  [TS_theta_RAD] -> Scope1/1, Product1/1
  [TS_ax] -> Selector1/1
  Product1/1 -> [TS_SIGNED_theta_RAD]
  Selector1/1 -> Product1/2
  PS-Simulink Converter7/1 -> [TS_theta_RAD]  "ang_wrt_W"
  PS-Simulink Converter8/1 -> [TS_ax]  "TS_ax"
  [TS_SIGNED_theta_RAD] -> Radians to Degrees/1
  PS-Simulink Converter5/1 -> Bus Creator/2  "omega_Z_degs_psec"
  connections:
  Transform Sensor/RConn1 -- Graphic1/RConn1 -- Graphic/RConn1 -- P/RConn1
  Transform Sensor/LConn1 -- World Frame/RConn1
  PS-Simulink Converter4/LConn1 -- Transform Sensor/RConn8
  PS-Simulink Converter2/LConn1 -- Transform Sensor/RConn7
  PS-Simulink Converter3/LConn1 -- Transform Sensor/RConn6
  PS-Simulink Converter1/LConn1 -- Transform Sensor/RConn5
  Transform Sensor/RConn2 -- PS-Simulink Converter7/LConn1
  PS-Simulink Converter8/LConn1 -- Transform Sensor/RConn3
  Transform Sensor/RConn4 -- PS-Simulink Converter5/LConn1

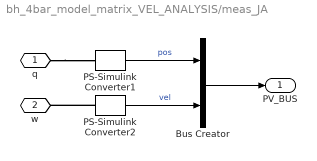
== system bh_4bar_model_matrix_VEL_ANALYSIS/meas_JA ==
  Bus Creator : BusCreator  Inputs=2
  PS-Simulink Converter1 : nesl_utility/PS-Simulink Converter  PhysicalDomain=network_engine_domain  SubClassName=ps_output  LeftPortType=input  RightPortType=output  PseudoPeriodic=off  Frequencies=[]  Unit=deg  AffineConversion=off
  PS-Simulink Converter2 : nesl_utility/PS-Simulink Converter  PhysicalDomain=network_engine_domain  SubClassName=ps_output  LeftPortType=input  RightPortType=output  PseudoPeriodic=off  Frequencies=[]  Unit=deg/s  AffineConversion=off
  q : PMIOPort  Side=Left
  w : PMIOPort  Port=2  Side=Left
  PV_BUS : Outport  VectorParamsAs1DForOutWhenUnconnected=off
  wires:
  PS-Simulink Converter2/1 -> Bus Creator/2  "vel"
  PS-Simulink Converter1/1 -> Bus Creator/1  "pos"
  Bus Creator/1 -> PV_BUS/1
  connections:
  q/RConn1 -- PS-Simulink Converter1/LConn1
  PS-Simulink Converter2/LConn1 -- w/RConn1

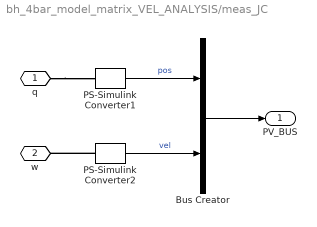
== system bh_4bar_model_matrix_VEL_ANALYSIS/meas_JC ==
  Bus Creator : BusCreator  Inputs=2
  PS-Simulink Converter1 : nesl_utility/PS-Simulink Converter  PhysicalDomain=network_engine_domain  SubClassName=ps_output  LeftPortType=input  RightPortType=output  PseudoPeriodic=off  Frequencies=[]  Unit=deg  AffineConversion=off
      settings: AttributesFormatString=UNITS=%<Unit>
  PS-Simulink Converter2 : nesl_utility/PS-Simulink Converter  PhysicalDomain=network_engine_domain  SubClassName=ps_output  LeftPortType=input  RightPortType=output  PseudoPeriodic=off  Frequencies=[]  Unit=deg/s  AffineConversion=off
      settings: AttributesFormatString=UNITS=%<Unit>
  q : PMIOPort  Side=Left
  w : PMIOPort  Port=2  Side=Left
  PV_BUS : Outport  VectorParamsAs1DForOutWhenUnconnected=off
  wires:
  PS-Simulink Converter2/1 -> Bus Creator/2  "vel"
  PS-Simulink Converter1/1 -> Bus Creator/1  "pos"
  Bus Creator/1 -> PV_BUS/1
  connections:
  q/RConn1 -- PS-Simulink Converter1/LConn1
  PS-Simulink Converter2/LConn1 -- w/RConn1

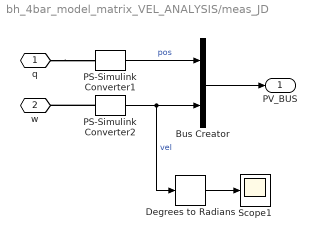
== system bh_4bar_model_matrix_VEL_ANALYSIS/meas_JD ==
  Bus Creator : BusCreator  Inputs=2
  Degrees to Radians : simulink_extras/Transformations/Degrees to Radians
  PS-Simulink Converter1 : nesl_utility/PS-Simulink Converter  PhysicalDomain=network_engine_domain  SubClassName=ps_output  LeftPortType=input  RightPortType=output  PseudoPeriodic=off  Frequencies=[]  Unit=deg  AffineConversion=off
  PS-Simulink Converter2 : nesl_utility/PS-Simulink Converter  PhysicalDomain=network_engine_domain  SubClassName=ps_output  LeftPortType=input  RightPortType=output  PseudoPeriodic=off  Frequencies=[]  Unit=deg/s  AffineConversion=off
  Scope1 : Scope
  q : PMIOPort  Side=Left
  w : PMIOPort  Port=2  Side=Left
  PV_BUS : Outport  VectorParamsAs1DForOutWhenUnconnected=off
  wires:
  PS-Simulink Converter2/1 -> Degrees to Radians/1, Bus Creator/2  "vel"
  PS-Simulink Converter1/1 -> Bus Creator/1  "pos"
  Bus Creator/1 -> PV_BUS/1
  Degrees to Radians/1 -> Scope1/1
  connections:
  q/RConn1 -- PS-Simulink Converter1/LConn1
  PS-Simulink Converter2/LConn1 -- w/RConn1
